simulink model "ATOM_simple_planning_2WS"  (R2026a)
settings: Solver=ode4  StopTime=15  FixedStep=0.01
model workspace (MAT data in the model file):
  vehicle.param.wheel_radius = 0.313
  vehicle.param.wheel_width = 0.235
  vehicle.param.wheel_base = 2
  vehicle.param.wheel_tread = 1.9
  vehicle.param.front_overhang = 0.46
  vehicle.param.rear_overhang = 0.46
  vehicle.param.left_overhang = 0.128
  vehicle.param.right_overhang = 0.128
  vehicle.param.vehicle_height = 1.8
  vehicle.param.max_steer_angle = 0.7
  vehicle.sim.vehicle_model_type = "DELAY_STEER_ACC_GEARED"
  vehicle.sim.initialize_source = "INITIAL_POSE_TOPIC"
  vehicle.sim.timer_sampling_time_ms = 25
  vehicle.sim.add_measurement_noise = 0
  vehicle.sim.vel_lim = 50
  vehicle.sim.vel_rate_lim = 7
  vehicle.sim.steer_lim = 1
  vehicle.sim.steer_rate_lim = 5
  vehicle.sim.acc_time_delay = 0.1
  vehicle.sim.acc_time_constant = 0.1
  vehicle.sim.steer_time_delay = 0.24
  vehicle.sim.steer_time_constant = 0.27
  vehicle.sim.x_stddev = 0.0001
  vehicle.sim.y_stddev = 0.0001
  vehicle.sim.steer_dead_band = 0
  vehicle.sim.steer_bias = 0
  vehicle.sim.debug_acc_scaling_factor = 1
  vehicle.sim.debug_steer_scaling_factor = 1
undefined symbols (not defined in the file or in its folder): planning_validator, stanley, velocity_smoother
(part 1 of 4)
settings Model: SimulationMode=accelerator  PacingRate=1000  Creator=andrea-ricetti  LastModifiedBy=andrea-ricetti

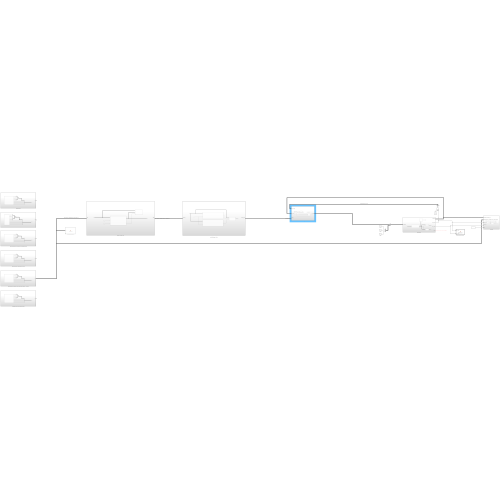
[thumbnail: Simulink's stored preview of the top-level diagram]
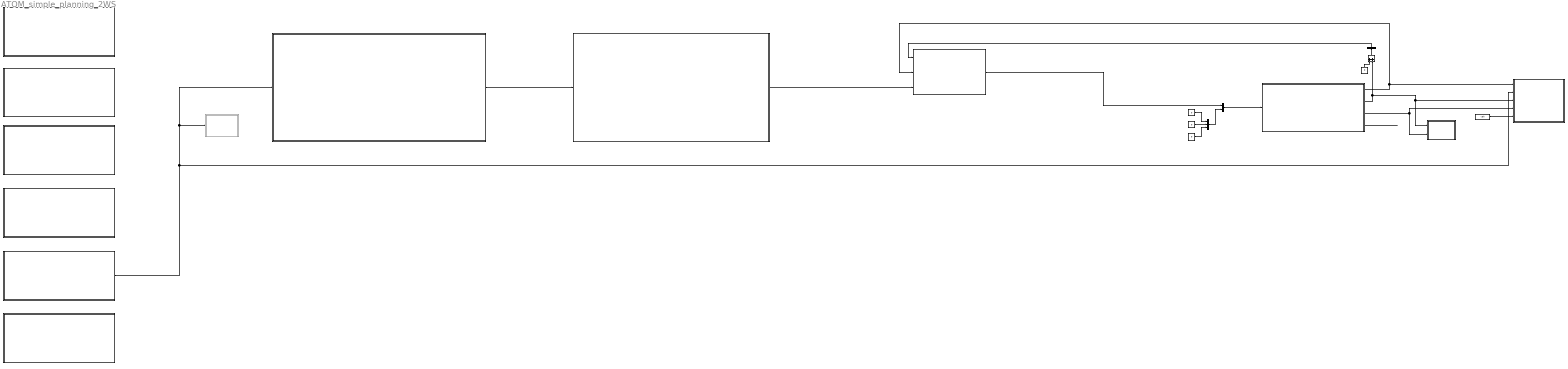
== system ATOM_simple_planning_2WS ==
  Add : Sum
  Bus Creator : BusCreator  Inputs=2  OutDataTypeStr=Bus: ControlCMDBus
      settings: InheritFromInputs=off
  Bus Creator2 : BusCreator  Inputs=3  OutDataTypeStr=Bus: LongitudinalBus
      settings: InheritFromInputs=off
  Bus Creator3 : BusCreator  Inputs=1  OutDataTypeStr=Bus: SteeringBus
      settings: InheritFromInputs=off
  Demanded trajectory generation: 90° left turn : Subsystem
  Demanded trajectory generation: 90° left turn critical for 2WS --> R = 2.5 m : Subsystem
  Demanded trajectory generation: Serpentine : Subsystem
  Demanded trajectory generation: Sinusoid 50m wavelength : Subsystem
  Demanded trajectory generation: smooth Parabola : Subsystem
  From Workspace1 : FromWorkspace  VariableName=veh
  Jerk : Constant  Value=0
  Lateral run() : Subsystem
  Plot demanded trajectory : MATLAB Function  Commented=on  TreatAsAtomicUnit=on
  Plot front/rear steer status : MATLAB Function  TreatAsAtomicUnit=on
  Plot vehicle : Subsystem
  Straight trajectory : Subsystem
  Vehicle Model : Subsystem
  acc : Constant  Value=0
  steer_bias : Constant  Value=0
  trajectory_checker plugin - planning_validator_node : Subsystem
  vel : Constant  Value=0
  velocity_smoother_node : Subsystem
  wires:
  Bus Creator2/1 -> Bus Creator/2
  vel/1 -> Bus Creator2/1
  acc/1 -> Bus Creator2/2
  Jerk/1 -> Bus Creator2/3
  Bus Creator/1 -> Vehicle Model/1(command)
  Vehicle Model/1(kinematic) -> Lateral run()/2(ego_pose), Plot vehicle/1(localization/kinematic_state)  "/localization/kinematic_state"
  Vehicle Model/3(steer_rear) -> Plot vehicle/4(steer_rear), Plot front/rear steer status/2(rear_steer)
  Demanded trajectory generation: 90° left turn critical for 2WS --> R = 2.5 m/1(traj) -> Plot vehicle/2(planning/scenario_planning/scenario_selector/trajectory), velocity_smoother_node/1(input), Plot demanded trajectory/1(traj)  "/planning/scenario_planning/scenario_selector/trajectory"
  Vehicle Model/4(accel) -> ?  "/localization/acceleration"
  velocity_smoother_node/1(output) -> trajectory_checker plugin - planning_validator_node/1(trajectory)  "/planning/scenario_planning/velocity_smoother/trajectory"
  trajectory_checker plugin - planning_validator_node/1(trajectory_out) -> Lateral run()/3(ref_traj)  "/planning/trajectory"
  Bus Creator3/1 -> Lateral run()/1(curr_steering)  "/vehicle/status/steering_status"
  Add/1 -> Bus Creator3/1
  steer_bias/1 -> Add/1
  Vehicle Model/2(steer_front) -> Add/2, Plot vehicle/3(steer_front), Plot front/rear steer status/1(front_steer)
  From Workspace1/1 -> Plot vehicle/5(veh)
  Lateral run()/1(ctrl_cmd) -> Bus Creator/1

== system ATOM_simple_planning_2WS/Demanded trajectory generation: 90° left turn ==
  Bus Creator3 : BusCreator  Inputs=3  OutDataTypeStr=Bus: PointBusN
  Bus Creator4 : BusCreator  Inputs=4  OutDataTypeStr=Bus: QuaternionBusN
  Bus Creator5 : BusCreator  Inputs=2  OutDataTypeStr=Bus: PoseBusN
      settings: InheritFromInputs=off
  Bus Creator6 : BusCreator  Inputs=7  OutDataTypeStr=Bus: TrajectoryDataBus
      settings: InheritFromInputs=off
  Trajectory Generator: 90° left turn : MATLAB Function  TreatAsAtomicUnit=on
  traj : Outport
  wires:
  Bus Creator6/1 -> traj/1
  Bus Creator3/1 -> Bus Creator5/1
  Trajectory Generator: 90° left turn/13(rear_wheel_angle_rad) -> Bus Creator6/7
  Bus Creator5/1 -> Bus Creator6/1
  Trajectory Generator: 90° left turn/8(longitudinal_velocity_mps) -> Bus Creator6/2
  Trajectory Generator: 90° left turn/3(z) -> Bus Creator3/3
  Trajectory Generator: 90° left turn/4(qx) -> Bus Creator4/1
  Trajectory Generator: 90° left turn/9(lateral_velocity_mps) -> Bus Creator6/3
  Trajectory Generator: 90° left turn/10(acceleration_mps2) -> Bus Creator6/4
  Trajectory Generator: 90° left turn/5(qy) -> Bus Creator4/2
  Trajectory Generator: 90° left turn/1(x) -> Bus Creator3/1
  Trajectory Generator: 90° left turn/2(y) -> Bus Creator3/2
  Trajectory Generator: 90° left turn/7(qw) -> Bus Creator4/4
  Trajectory Generator: 90° left turn/6(qz) -> Bus Creator4/3
  Trajectory Generator: 90° left turn/12(front_wheel_angle_rad) -> Bus Creator6/6
  Bus Creator4/1 -> Bus Creator5/2
  Trajectory Generator: 90° left turn/11(heading_rate_rps) -> Bus Creator6/5

== system ATOM_simple_planning_2WS/Demanded trajectory generation: 90° left turn critical for 2WS --> R = 2.5 m ==
  Bus Creator3 : BusCreator  Inputs=3  OutDataTypeStr=Bus: PointBusN
  Bus Creator4 : BusCreator  Inputs=4  OutDataTypeStr=Bus: QuaternionBusN
  Bus Creator5 : BusCreator  Inputs=2  OutDataTypeStr=Bus: PoseBusN
      settings: InheritFromInputs=off
  Bus Creator6 : BusCreator  Inputs=7  OutDataTypeStr=Bus: TrajectoryDataBus
      settings: InheritFromInputs=off
  Trajectory Generator: 90° left turn critical for 2WS : MATLAB Function  TreatAsAtomicUnit=on
  traj : Outport
  wires:
  Bus Creator6/1 -> traj/1
  Bus Creator3/1 -> Bus Creator5/1
  Trajectory Generator: 90° left turn critical for 2WS/13(rear_wheel_angle_rad) -> Bus Creator6/7
  Bus Creator5/1 -> Bus Creator6/1
  Trajectory Generator: 90° left turn critical for 2WS/8(longitudinal_velocity_mps) -> Bus Creator6/2
  Trajectory Generator: 90° left turn critical for 2WS/3(z) -> Bus Creator3/3
  Trajectory Generator: 90° left turn critical for 2WS/4(qx) -> Bus Creator4/1
  Trajectory Generator: 90° left turn critical for 2WS/9(lateral_velocity_mps) -> Bus Creator6/3
  Trajectory Generator: 90° left turn critical for 2WS/10(acceleration_mps2) -> Bus Creator6/4
  Trajectory Generator: 90° left turn critical for 2WS/5(qy) -> Bus Creator4/2
  Trajectory Generator: 90° left turn critical for 2WS/1(x) -> Bus Creator3/1
  Trajectory Generator: 90° left turn critical for 2WS/2(y) -> Bus Creator3/2
  Trajectory Generator: 90° left turn critical for 2WS/7(qw) -> Bus Creator4/4
  Trajectory Generator: 90° left turn critical for 2WS/6(qz) -> Bus Creator4/3
  Trajectory Generator: 90° left turn critical for 2WS/12(front_wheel_angle_rad) -> Bus Creator6/6
  Bus Creator4/1 -> Bus Creator5/2
  Trajectory Generator: 90° left turn critical for 2WS/11(heading_rate_rps) -> Bus Creator6/5

== system ATOM_simple_planning_2WS/Demanded trajectory generation: Serpentine ==
  Bus Creator3 : BusCreator  Inputs=3  OutDataTypeStr=Bus: PointBusN
  Bus Creator4 : BusCreator  Inputs=4  OutDataTypeStr=Bus: QuaternionBusN
  Bus Creator5 : BusCreator  Inputs=2  OutDataTypeStr=Bus: PoseBusN
      settings: InheritFromInputs=off
  Bus Creator6 : BusCreator  Inputs=7  OutDataTypeStr=Bus: TrajectoryDataBus
      settings: InheritFromInputs=off
  Trajectory Generator: 90° left turn critical for 2WS : MATLAB Function  TreatAsAtomicUnit=on
  traj : Outport
  wires:
  Bus Creator6/1 -> traj/1
  Bus Creator3/1 -> Bus Creator5/1
  Trajectory Generator: 90° left turn critical for 2WS/13(rear_wheel_angle_rad) -> Bus Creator6/7
  Bus Creator5/1 -> Bus Creator6/1
  Trajectory Generator: 90° left turn critical for 2WS/8(longitudinal_velocity_mps) -> Bus Creator6/2
  Trajectory Generator: 90° left turn critical for 2WS/3(z) -> Bus Creator3/3
  Trajectory Generator: 90° left turn critical for 2WS/4(qx) -> Bus Creator4/1
  Trajectory Generator: 90° left turn critical for 2WS/9(lateral_velocity_mps) -> Bus Creator6/3
  Trajectory Generator: 90° left turn critical for 2WS/10(acceleration_mps2) -> Bus Creator6/4
  Trajectory Generator: 90° left turn critical for 2WS/5(qy) -> Bus Creator4/2
  Trajectory Generator: 90° left turn critical for 2WS/1(x) -> Bus Creator3/1
  Trajectory Generator: 90° left turn critical for 2WS/2(y) -> Bus Creator3/2
  Trajectory Generator: 90° left turn critical for 2WS/7(qw) -> Bus Creator4/4
  Trajectory Generator: 90° left turn critical for 2WS/6(qz) -> Bus Creator4/3
  Trajectory Generator: 90° left turn critical for 2WS/12(front_wheel_angle_rad) -> Bus Creator6/6
  Bus Creator4/1 -> Bus Creator5/2
  Trajectory Generator: 90° left turn critical for 2WS/11(heading_rate_rps) -> Bus Creator6/5

== system ATOM_simple_planning_2WS/Demanded trajectory generation: Sinusoid 50m wavelength ==
  Bus Creator3 : BusCreator  Inputs=3  OutDataTypeStr=Bus: PointBusN
  Bus Creator4 : BusCreator  Inputs=4  OutDataTypeStr=Bus: QuaternionBusN
  Bus Creator5 : BusCreator  Inputs=2  OutDataTypeStr=Bus: PoseBusN
      settings: InheritFromInputs=off
  Bus Creator6 : BusCreator  Inputs=7  OutDataTypeStr=Bus: TrajectoryDataBus
      settings: InheritFromInputs=off
  Trajectory Generator: sinusoid : MATLAB Function  TreatAsAtomicUnit=on
  traj : Outport
  wires:
  Bus Creator6/1 -> traj/1
  Bus Creator3/1 -> Bus Creator5/1
  Trajectory Generator: sinusoid/13(rear_wheel_angle_rad) -> Bus Creator6/7
  Bus Creator5/1 -> Bus Creator6/1
  Trajectory Generator: sinusoid/8(longitudinal_velocity_mps) -> Bus Creator6/2
  Trajectory Generator: sinusoid/3(z) -> Bus Creator3/3
  Trajectory Generator: sinusoid/4(qx) -> Bus Creator4/1
  Trajectory Generator: sinusoid/9(lateral_velocity_mps) -> Bus Creator6/3
  Trajectory Generator: sinusoid/10(acceleration_mps2) -> Bus Creator6/4
  Trajectory Generator: sinusoid/5(qy) -> Bus Creator4/2
  Trajectory Generator: sinusoid/1(x) -> Bus Creator3/1
  Trajectory Generator: sinusoid/2(y) -> Bus Creator3/2
  Trajectory Generator: sinusoid/7(qw) -> Bus Creator4/4
  Trajectory Generator: sinusoid/6(qz) -> Bus Creator4/3
  Trajectory Generator: sinusoid/12(front_wheel_angle_rad) -> Bus Creator6/6
  Bus Creator4/1 -> Bus Creator5/2
  Trajectory Generator: sinusoid/11(heading_rate_rps) -> Bus Creator6/5

== system ATOM_simple_planning_2WS/Demanded trajectory generation: smooth Parabola ==
  Bus Creator3 : BusCreator  Inputs=3  OutDataTypeStr=Bus: PointBusN
  Bus Creator4 : BusCreator  Inputs=4  OutDataTypeStr=Bus: QuaternionBusN
  Bus Creator5 : BusCreator  Inputs=2  OutDataTypeStr=Bus: PoseBusN
      settings: InheritFromInputs=off
  Bus Creator6 : BusCreator  Inputs=7  OutDataTypeStr=Bus: TrajectoryDataBus
      settings: InheritFromInputs=off
  Smoothed Parabola trajectory : MATLAB Function  TreatAsAtomicUnit=on
  traj : Outport
  wires:
  Smoothed Parabola trajectory/5(qy) -> Bus Creator4/2
  Smoothed Parabola trajectory/6(qz) -> Bus Creator4/3
  Smoothed Parabola trajectory/11(heading_rate_rps) -> Bus Creator6/5
  Bus Creator5/1 -> Bus Creator6/1
  Bus Creator6/1 -> traj/1
  Smoothed Parabola trajectory/3(z) -> Bus Creator3/3
  Bus Creator4/1 -> Bus Creator5/2
  Smoothed Parabola trajectory/8(longitudinal_velocity_mps) -> Bus Creator6/2
  Smoothed Parabola trajectory/4(qx) -> Bus Creator4/1
  Smoothed Parabola trajectory/13(rear_wheel_angle_rad) -> Bus Creator6/7
  Smoothed Parabola trajectory/7(qw) -> Bus Creator4/4
  Smoothed Parabola trajectory/1(x) -> Bus Creator3/1
  Smoothed Parabola trajectory/2(y) -> Bus Creator3/2
  Bus Creator3/1 -> Bus Creator5/1
  Smoothed Parabola trajectory/12(front_wheel_angle_rad) -> Bus Creator6/6
  Smoothed Parabola trajectory/10(acceleration_mps2) -> Bus Creator6/4
  Smoothed Parabola trajectory/9(lateral_velocity_mps) -> Bus Creator6/3

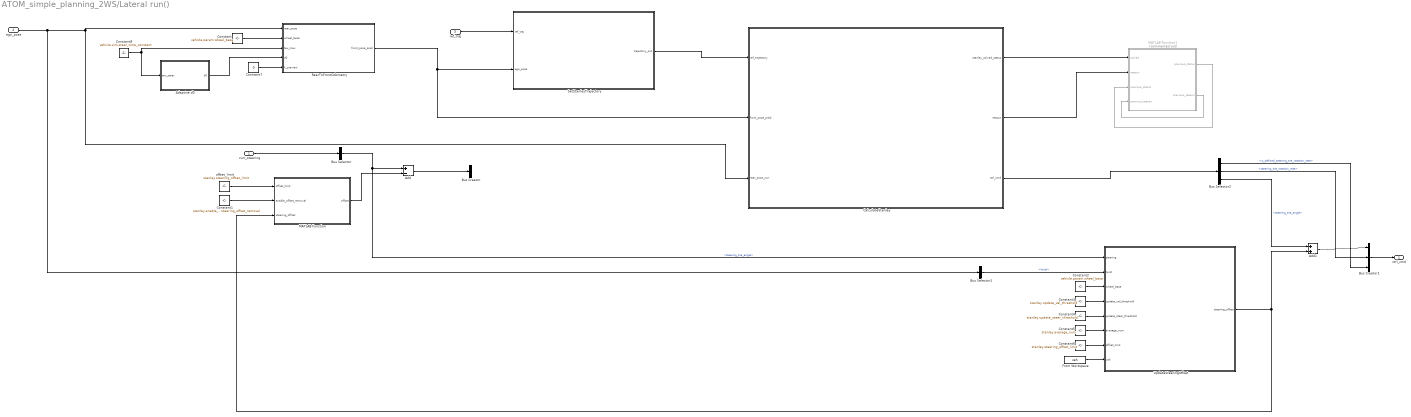
== system ATOM_simple_planning_2WS/Lateral run() ==
  curr_steering : Inport
  ego_pose : Inport  Port=2
  ref_traj : Inport  Port=3
  Adaptive d0 : MATLAB Function  TreatAsAtomicUnit=on
  Add : Sum  Inputs=+-
  Add1 : Sum
  Bus Creator : BusCreator  Inputs=1  OutDataTypeStr=Bus: SteeringBus
      settings: InheritFromInputs=off
  Bus Creator1 : BusCreator  Inputs=3  OutDataTypeStr=Bus: LateralBus
      settings: InheritFromInputs=off
  Bus Selector : BusSelector  OutputSignals=steering_tire_angle
  Bus Selector1 : BusSelector  OutputSignals=twist
  Bus Selector2 : BusSelector  OutputSignals=is_defined_steering_tire_rotation_rate,steering_tire_rotation_rate,steering_tire_angle
  CalculateStanley : Subsystem
  Constant : Constant  Value=vehicle.param.wheel_base
  Constant1 : Constant  Value=stanley.enable_auto_steering_offset_removal
  Constant2 : Constant  Value=vehicle.param.wheel_base
  Constant3 : Constant  Value=stanley.update_vel_threshold
  Constant4 : Constant  Value=stanley.update_steer_threshold
  Constant5 : Constant  Value=stanley.average_num
  Constant6 : Constant  Value=stanley.steering_offset_limit
  Constant7 : Constant  Value=0
  Constant8 : Constant  Value=vehicle.sim.steer_time_constant
  From Workspace : FromWorkspace  VariableName=veh
  MATLAB Function : MATLAB Function  TreatAsAtomicUnit=on
  MATLAB Function1 : MATLAB Function  Commented=on  TreatAsAtomicUnit=on
  RearToFrontOdometry : MATLAB Function  TreatAsAtomicUnit=on
  SetStanleyTrajectory : Subsystem
  UpdateSteeringOffset : MATLAB Function  TreatAsAtomicUnit=on
  offset_limit : Constant  Value=stanley.steering_offset_limit
  ctrl_cmd : Outport
  wires:
  ego_pose/1 -> Bus Selector1/1, CalculateStanley/3(rear_pose_curr), RearToFrontOdometry/1(rear_pose)
  Constant/1 -> RearToFrontOdometry/2(wheel_base)
  RearToFrontOdometry/1(front_pose_pred) -> CalculateStanley/2(front_pose_pred), SetStanleyTrajectory/2(ego_pose)
  curr_steering/1 -> Bus Selector/1
  offset_limit/1 -> MATLAB Function/1(offset_limit)
  Constant1/1 -> MATLAB Function/2(enable_offset_removal)
  Add/1 -> Bus Creator/1
  Bus Selector/1 -> UpdateSteeringOffset/1(steering), Add/1  "<steering_tire_angle>"
  ref_traj/1 -> SetStanleyTrajectory/1(ref_traj)
  SetStanleyTrajectory/1(trajectory_out) -> CalculateStanley/1(ref_trajectory)
  CalculateStanley/1(stanley_solved_status) -> MATLAB Function1/1(solved)
  CalculateStanley/2(reason) -> MATLAB Function1/2(reason)
  MATLAB Function1/2(previous_reason) -> MATLAB Function1/4("previous_reason ")
  MATLAB Function1/1(previous_status) -> MATLAB Function1/3("previous_status ")
  Bus Selector1/1 -> UpdateSteeringOffset/2(twist)  "<twist>"
  Constant2/1 -> UpdateSteeringOffset/3(wheel_base)
  Constant3/1 -> UpdateSteeringOffset/4(update_vel_threshold)
  Constant5/1 -> UpdateSteeringOffset/6(average_num)
  Constant4/1 -> UpdateSteeringOffset/5(update_steer_threshold)
  Constant6/1 -> UpdateSteeringOffset/7(offset_limit)
  From Workspace/1 -> UpdateSteeringOffset/8(veh)
  CalculateStanley/3(ctrl_cmd) -> Bus Selector2/1
  Bus Selector2/3 -> Add1/1  "<steering_tire_angle>"
  Add1/1 -> Bus Creator1/1
  Bus Selector2/1 -> Bus Creator1/3  "<is_defined_steering_tire_rotation_rate>"
  Bus Selector2/2 -> Bus Creator1/2  "<steering_tire_rotation_rate>"
  Bus Creator1/1 -> ctrl_cmd/1
  MATLAB Function/1(offset) -> Add/2
  UpdateSteeringOffset/1(steering_offset) -> MATLAB Function/3(steering_offset), Add1/2
  Constant8/1 -> Adaptive d0/1(tau_steer), RearToFrontOdometry/3(tau_max)
  Adaptive d0/1(d0) -> RearToFrontOdometry/4(d0)
  Constant7/1 -> RearToFrontOdometry/5(k_preview)

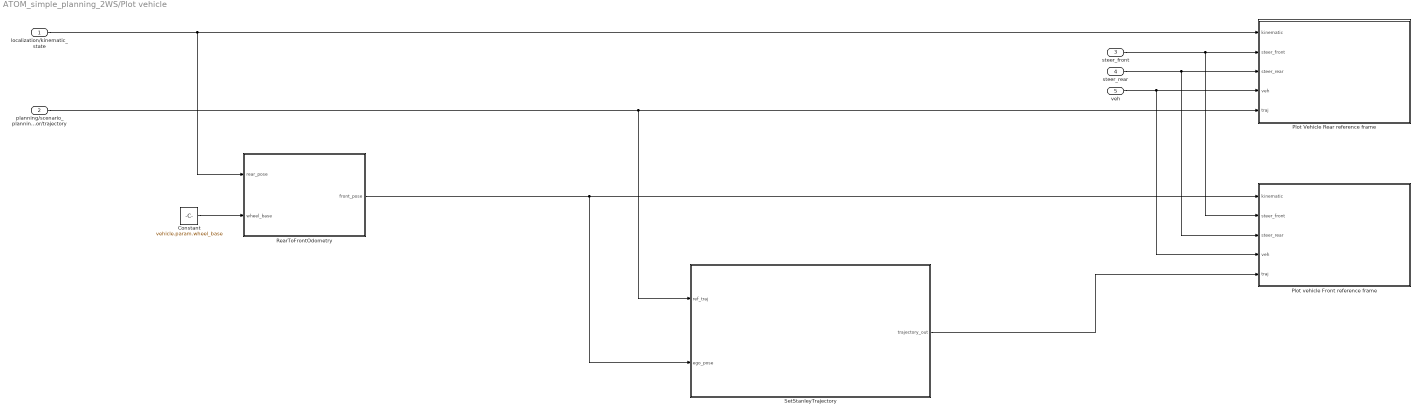
== system ATOM_simple_planning_2WS/Plot vehicle ==
  localization/kinematic_state : Inport
  planning/scenario_planning/scenario_selector/trajectory : Inport  Port=2
  steer_front : Inport  Port=3
  steer_rear : Inport  Port=4
  veh : Inport  Port=5
  Constant : Constant  Value=vehicle.param.wheel_base
  Plot Vehicle Rear reference frame : MATLAB Function  TreatAsAtomicUnit=on
  Plot vehicle Front reference frame : MATLAB Function  TreatAsAtomicUnit=on
  RearToFrontOdometry : MATLAB Function  TreatAsAtomicUnit=on
  SetStanleyTrajectory : Subsystem
  wires:
  steer_rear/1 -> Plot vehicle Front reference frame/3(steer_rear), Plot Vehicle Rear reference frame/3(steer_rear)
  veh/1 -> Plot vehicle Front reference frame/4(veh), Plot Vehicle Rear reference frame/4(veh)
  steer_front/1 -> Plot vehicle Front reference frame/2(steer_front), Plot Vehicle Rear reference frame/2(steer_front)
  Constant/1 -> RearToFrontOdometry/2(wheel_base)
  localization/kinematic_state/1 -> Plot Vehicle Rear reference frame/1(kinematic), RearToFrontOdometry/1(rear_pose)
  planning/scenario_planning/scenario_selector/trajectory/1 -> SetStanleyTrajectory/1(ref_traj), Plot Vehicle Rear reference frame/5(traj)
  RearToFrontOdometry/1(front_pose) -> SetStanleyTrajectory/2(ego_pose), Plot vehicle Front reference frame/1(kinematic)
  SetStanleyTrajectory/1(trajectory_out) -> Plot vehicle Front reference frame/5(traj)

== system ATOM_simple_planning_2WS/Straight trajectory ==
  Bus Creator3 : BusCreator  Inputs=3  OutDataTypeStr=Bus: PointBusN
  Bus Creator4 : BusCreator  Inputs=4  OutDataTypeStr=Bus: QuaternionBusN
  Bus Creator5 : BusCreator  Inputs=2  OutDataTypeStr=Bus: PoseBusN
      settings: InheritFromInputs=off
  Bus Creator6 : BusCreator  Inputs=7  OutDataTypeStr=Bus: TrajectoryDataBus
      settings: InheritFromInputs=off
  Trajectory Generator: straight : MATLAB Function  TreatAsAtomicUnit=on
  traj : Outport
  wires:
  Bus Creator6/1 -> traj/1
  Bus Creator3/1 -> Bus Creator5/1
  Trajectory Generator: straight/13(rear_wheel_angle_rad) -> Bus Creator6/7
  Bus Creator5/1 -> Bus Creator6/1
  Trajectory Generator: straight/8(longitudinal_velocity_mps) -> Bus Creator6/2
  Trajectory Generator: straight/3(z) -> Bus Creator3/3
  Trajectory Generator: straight/4(qx) -> Bus Creator4/1
  Trajectory Generator: straight/9(lateral_velocity_mps) -> Bus Creator6/3
  Trajectory Generator: straight/10(acceleration_mps2) -> Bus Creator6/4
  Trajectory Generator: straight/5(qy) -> Bus Creator4/2
  Trajectory Generator: straight/1(x) -> Bus Creator3/1
  Trajectory Generator: straight/2(y) -> Bus Creator3/2
  Trajectory Generator: straight/7(qw) -> Bus Creator4/4
  Trajectory Generator: straight/6(qz) -> Bus Creator4/3
  Trajectory Generator: straight/12(front_wheel_angle_rad) -> Bus Creator6/6
  Bus Creator4/1 -> Bus Creator5/2
  Trajectory Generator: straight/11(heading_rate_rps) -> Bus Creator6/5

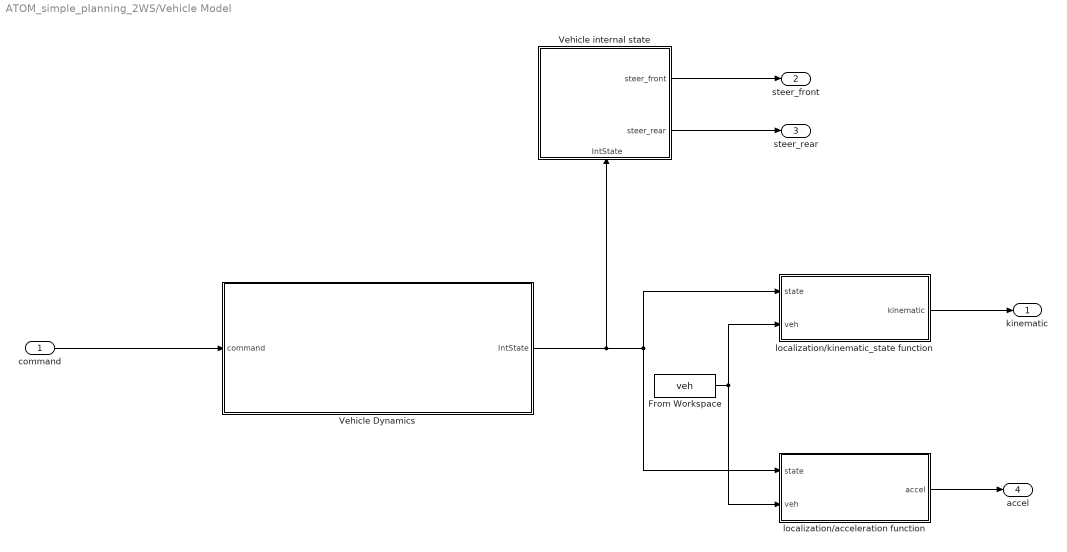
== system ATOM_simple_planning_2WS/Vehicle Model ==
  command : Inport
  From Workspace : FromWorkspace  VariableName=veh
  Vehicle Dynamics : Subsystem
  Vehicle internal state : Subsystem
      settings: PortSchema="{\"entries\":[{\"content\":{\"sides\":[{\"content\":{},\"type\":\"ConnectorPlacement.EquallySpacedRectSide\",\"uuid\":\"4a3566d2-c9ed-40f5-9383-803dea843249\"},{\"content\":{\"connectorIds\":[\"Out1\",\"Out2\"],\"side\":\"RIGHT\"},\"type\":\"ConnectorPlacement.EquallySpacedRectSide\",\"uuid\":\"38e6b545-4a7a-4953-bfc7-602e8f089057\"},{\"content\":{\"side\":\"TOP\"},\"type\":\"ConnectorPlacement.EquallySpacedRectSide\",\"uuid\":\"85394c7e-506c-43bc-a81e-512f61060685\"},{\"content\":{\"connectorIds\":[\"In1\"],\"side\":\"BOTTOM\"},\"type\":\"ConnectorPlacement.EquallySpacedRectSide\",\"uuid\":\"97da4b67-3c43-4e7d-b3d8-7f85e7f15c39\"}]},\"type\":\"ConnectorPlacement.EquallySpacedConnector\",\"uuid\":\"d0ddb274-13a9-46fc-8356-ac8c2bb4db82\"}],\"packageUris\":[\"http://schema.mathworks.com/mf0/Connector/R2020b\"],\"version\":\"1.0\"}"
  localization/acceleration function : MATLAB Function  TreatAsAtomicUnit=on
  localization/kinematic_state function : MATLAB Function  TreatAsAtomicUnit=on
  kinematic : Outport
  steer_front : Outport  Port=2
  steer_rear : Outport  Port=3
  accel : Outport  Port=4
  wires:
  From Workspace/1 -> localization/acceleration function/2(veh), localization/kinematic_state function/2(veh)
  Vehicle Dynamics/1(IntState) -> localization/kinematic_state function/1(state), localization/acceleration function/1(state), Vehicle internal state/1(IntState)
  Vehicle internal state/2(steer_rear) -> steer_rear/1
  command/1 -> Vehicle Dynamics/1(command)
  localization/kinematic_state function/1(kinematic) -> kinematic/1
  Vehicle internal state/1(steer_front) -> steer_front/1
  localization/acceleration function/1(accel) -> accel/1

== system ATOM_simple_planning_2WS/trajectory_checker plugin - planning_validator_node ==
  trajectory : Inport
  From Workspace2 : FromWorkspace  VariableName=veh
  HandleInvalidTrajectory - handling_type == default (case 0) : MATLAB Function  TreatAsAtomicUnit=on
  check_valid_steering : Subsystem
  check_valid_steering_rate : Subsystem
  trajectory_out : Outport
  wires:
  From Workspace2/1 -> check_valid_steering_rate/2(veh), check_valid_steering/2(veh)
  trajectory/1 -> check_valid_steering_rate/1(trajectory), HandleInvalidTrajectory - handling_type == default (case 0)/1(trajectory_in), check_valid_steering/1(trajectory)
  check_valid_steering/1(is_valid_steering) -> HandleInvalidTrajectory - handling_type == default (case 0)/2(is_valid_steering)
  check_valid_steering_rate/1(is_valid_steering_rate) -> HandleInvalidTrajectory - handling_type == default (case 0)/3(is_valid_steering_rate)
  HandleInvalidTrajectory - handling_type == default (case 0)/1(trajectory_out) -> trajectory_out/1

== system ATOM_simple_planning_2WS/velocity_smoother_node ==
  input : Inport
  ApplySteeringRateLimit - velocity_smoother_node : Subsystem
  MATLAB Function : MATLAB Function  Commented=on  TreatAsAtomicUnit=on
  input_points_interval [m] : Constant  OutDataTypeStr=double
  use_resampling == false : Constant  Value=0  OutDataTypeStr=boolean
  output : Outport
  wires:
  use_resampling == false/1 -> ApplySteeringRateLimit - velocity_smoother_node/2(use_resampling)
  ApplySteeringRateLimit - velocity_smoother_node/2(curvature) -> MATLAB Function/3(curvature)
  input/1 -> MATLAB Function/1(trajectory_input), ApplySteeringRateLimit - velocity_smoother_node/1(input From Trajecory topic --> TrajectoryPoints format)
  input_points_interval [m]/1 -> ApplySteeringRateLimit - velocity_smoother_node/3(input_points_interval)
  ApplySteeringRateLimit - velocity_smoother_node/1(output) -> output/1, MATLAB Function/2(trajectory_output)

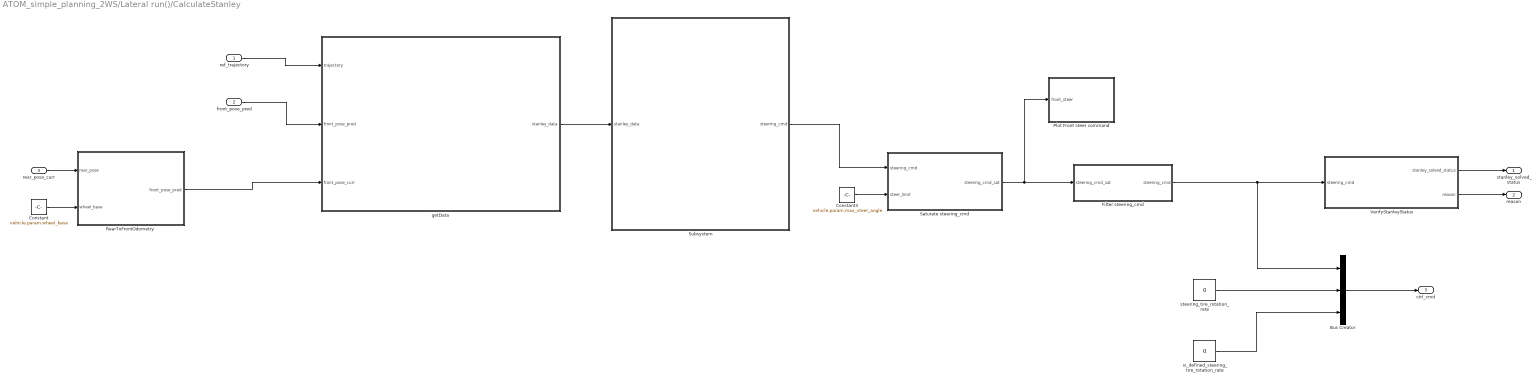
== system ATOM_simple_planning_2WS/Lateral run()/CalculateStanley ==
  ref_trajectory : Inport
  front_pose_pred : Inport  Port=2
  rear_pose_curr : Inport  Port=3
  Bus Creator : BusCreator  Inputs=3  OutDataTypeStr=Bus: LateralBus
      settings: InheritFromInputs=off
  Constant : Constant  Value=vehicle.param.wheel_base
  Constant3 : Constant  Value=vehicle.param.max_steer_angle
  Filter steering_cmd : MATLAB Function  TreatAsAtomicUnit=on
  Plot Front steer command : MATLAB Function  TreatAsAtomicUnit=on
  RearToFrontOdometry : MATLAB Function  TreatAsAtomicUnit=on
  Saturate steering_cmd : MATLAB Function  TreatAsAtomicUnit=on
  Subsystem : Subsystem
  VerifyStanleyStatus : MATLAB Function  TreatAsAtomicUnit=on
  getData : Subsystem
  is_defined_steering_tire_rotation_rate : Constant  Value=0  OutDataTypeStr=boolean
  steering_tire_rotation_rate : Constant  Value=0
  stanley_solved_status : Outport
  reason : Outport  Port=2
  ctrl_cmd : Outport  Port=3
  wires:
  ref_trajectory/1 -> getData/1(trajectory)
  front_pose_pred/1 -> getData/2(front_pose_pred)
  Constant3/1 -> Saturate steering_cmd/2(steer_limit)
  Saturate steering_cmd/1(steering_cmd_sat) -> Plot Front steer command/1(front_steer), Filter steering_cmd/1(steering_cmd_sat)
  Filter steering_cmd/1(steering_cmd) -> VerifyStanleyStatus/1(steering_cmd), Bus Creator/1
  steering_tire_rotation_rate/1 -> Bus Creator/2
  is_defined_steering_tire_rotation_rate/1 -> Bus Creator/3
  Bus Creator/1 -> ctrl_cmd/1
  VerifyStanleyStatus/1(stanley_solved_status) -> stanley_solved_status/1
  VerifyStanleyStatus/2(reason) -> reason/1
  getData/1(stanley_data) -> Subsystem/1(stanley_data)
  Subsystem/1(steering_cmd) -> Saturate steering_cmd/1(steering_cmd)
  Constant/1 -> RearToFrontOdometry/2(wheel_base)
  rear_pose_curr/1 -> RearToFrontOdometry/1(rear_pose)
  RearToFrontOdometry/1(front_pose_pred) -> getData/3(front_pose_curr)

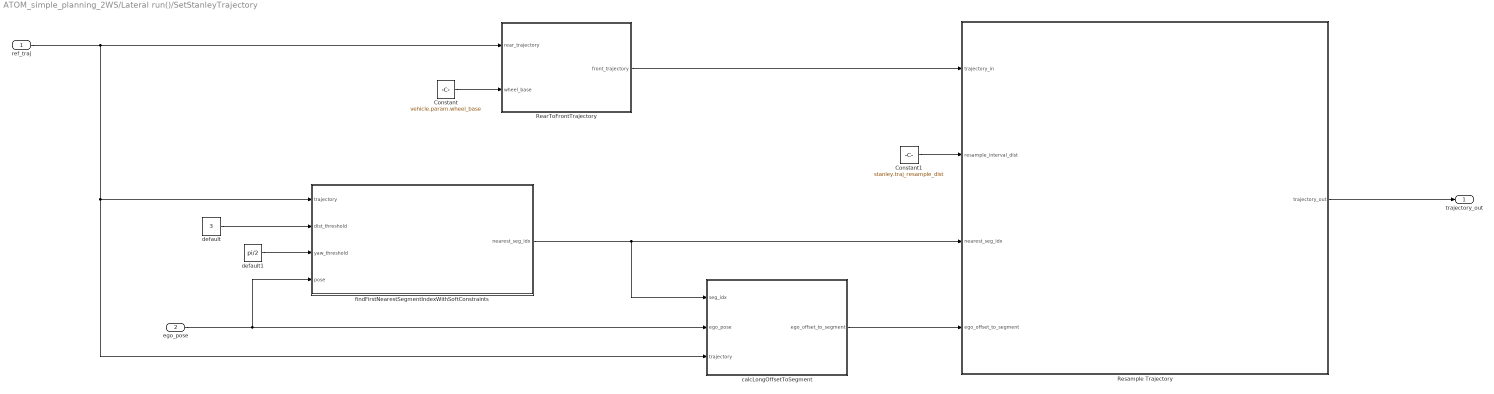
== system ATOM_simple_planning_2WS/Lateral run()/SetStanleyTrajectory ==
  ref_traj : Inport
  ego_pose : Inport  Port=2
  Constant : Constant  Value=vehicle.param.wheel_base
  Constant1 : Constant  Value=stanley.traj_resample_dist
  RearToFrontTrajectory : MATLAB Function  TreatAsAtomicUnit=on
  Resample Trajectory : MATLAB Function  TreatAsAtomicUnit=on
  calcLongOffsetToSegment : MATLAB Function  TreatAsAtomicUnit=on
  default : Constant  Value=3
  default1 : Constant  Value=pi/2
  findFirstNearestSegmentIndexWithSoftConstraints : MATLAB Function  TreatAsAtomicUnit=on
  trajectory_out : Outport
  wires:
  ref_traj/1 -> calcLongOffsetToSegment/3(trajectory), findFirstNearestSegmentIndexWithSoftConstraints/1(trajectory), RearToFrontTrajectory/1(rear_trajectory)
  Constant1/1 -> Resample Trajectory/2(resample_interval_dist)
  calcLongOffsetToSegment/1(ego_offset_to_segment) -> Resample Trajectory/4(ego_offset_to_segment)
  ego_pose/1 -> findFirstNearestSegmentIndexWithSoftConstraints/4(pose), calcLongOffsetToSegment/2(ego_pose)
  findFirstNearestSegmentIndexWithSoftConstraints/1(nearest_seg_idx) -> calcLongOffsetToSegment/1(seg_idx), Resample Trajectory/3(nearest_seg_idx)
  default/1 -> findFirstNearestSegmentIndexWithSoftConstraints/2(dist_threshold)
  default1/1 -> findFirstNearestSegmentIndexWithSoftConstraints/3(yaw_threshold)
  Resample Trajectory/1(trajectory_out) -> trajectory_out/1
  RearToFrontTrajectory/1(front_trajectory) -> Resample Trajectory/1(trajectory_in)
  Constant/1 -> RearToFrontTrajectory/2(wheel_base)

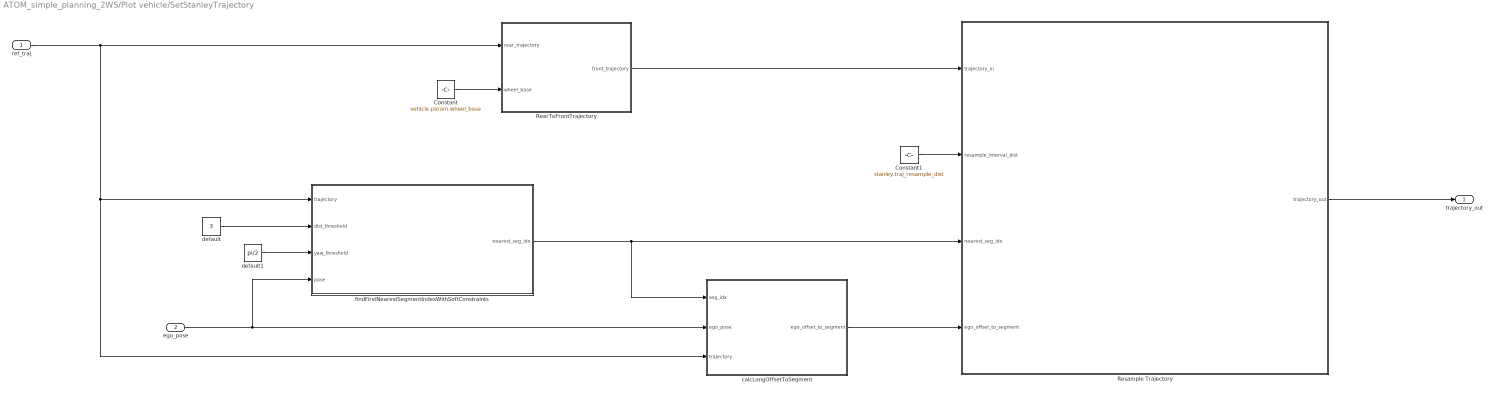
== system ATOM_simple_planning_2WS/Plot vehicle/SetStanleyTrajectory ==
  ref_traj : Inport
  ego_pose : Inport  Port=2
  Constant : Constant  Value=vehicle.param.wheel_base
  Constant1 : Constant  Value=stanley.traj_resample_dist
  RearToFrontTrajectory : MATLAB Function  TreatAsAtomicUnit=on
  Resample Trajectory : MATLAB Function  TreatAsAtomicUnit=on
  calcLongOffsetToSegment : MATLAB Function  TreatAsAtomicUnit=on
  default : Constant  Value=3
  default1 : Constant  Value=pi/2
  findFirstNearestSegmentIndexWithSoftConstraints : MATLAB Function  TreatAsAtomicUnit=on
  trajectory_out : Outport
  wires:
  ref_traj/1 -> calcLongOffsetToSegment/3(trajectory), findFirstNearestSegmentIndexWithSoftConstraints/1(trajectory), RearToFrontTrajectory/1(rear_trajectory)
  Constant1/1 -> Resample Trajectory/2(resample_interval_dist)
  calcLongOffsetToSegment/1(ego_offset_to_segment) -> Resample Trajectory/4(ego_offset_to_segment)
  ego_pose/1 -> findFirstNearestSegmentIndexWithSoftConstraints/4(pose), calcLongOffsetToSegment/2(ego_pose)
  findFirstNearestSegmentIndexWithSoftConstraints/1(nearest_seg_idx) -> calcLongOffsetToSegment/1(seg_idx), Resample Trajectory/3(nearest_seg_idx)
  default/1 -> findFirstNearestSegmentIndexWithSoftConstraints/2(dist_threshold)
  default1/1 -> findFirstNearestSegmentIndexWithSoftConstraints/3(yaw_threshold)
  Resample Trajectory/1(trajectory_out) -> trajectory_out/1
  RearToFrontTrajectory/1(front_trajectory) -> Resample Trajectory/1(trajectory_in)
  Constant/1 -> RearToFrontTrajectory/2(wheel_base)

== system ATOM_simple_planning_2WS/Vehicle Model/Vehicle Dynamics ==
  command : Inport
  From Workspace : FromWorkspace  VariableName=veh
  MATLAB Function : MATLAB Function  TreatAsAtomicUnit=on
  state integrator : Subsystem
  IntState : Outport
  wires:
  command/1 -> MATLAB Function/2(command)
  MATLAB Function/1(d_state) -> state integrator/1(d_state)  "d_state"
  state integrator/1(state) -> MATLAB Function/1(state), IntState/1
  From Workspace/1 -> MATLAB Function/3(veh)

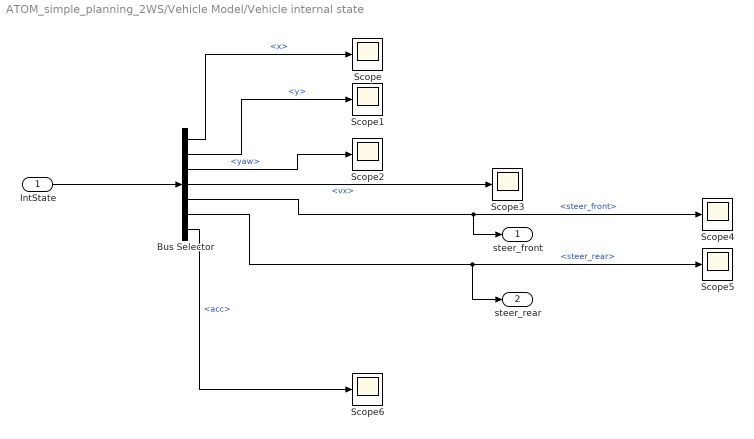
== system ATOM_simple_planning_2WS/Vehicle Model/Vehicle internal state ==
  IntState : Inport
  Bus Selector : BusSelector  OutputSignals=x,y,yaw,vx,steer_front,steer_rear,acc
  Scope{,1..6} (7 alike) : Scope
      Scope settings: ActiveDisplayYMinimum=-1  ActiveDisplayYMaximum=1
      Scope1 settings: ActiveDisplayYMinimum=-1  ActiveDisplayYMaximum=1
      Scope2 settings: ActiveDisplayYMinimum=-1  ActiveDisplayYMaximum=1  DataLoggingVariableName=ScopeData2
      Scope3 settings: ActiveDisplayYMinimum=-1  ActiveDisplayYMaximum=1  DataLoggingVariableName=ScopeData3
      Scope4 settings: ActiveDisplayYMinimum=-1  ActiveDisplayYMaximum=1  DataLoggingVariableName=ScopeData4
      Scope5 settings: ActiveDisplayYMinimum=-1  ActiveDisplayYMaximum=1  DataLoggingVariableName=ScopeData5
      Scope6 settings: ActiveDisplayYMinimum=-1  ActiveDisplayYMaximum=1  DataLoggingVariableName=ScopeData6
  steer_front : Outport
  steer_rear : Outport  Port=2
  wires:
  Bus Selector/2 -> Scope1/1  "<y>"
  Bus Selector/4 -> Scope3/1  "<vx>"
  Bus Selector/1 -> Scope/1  "<x>"
  Bus Selector/3 -> Scope2/1  "<yaw>"
  Bus Selector/7 -> Scope6/1  "<acc>"
  Bus Selector/5 -> steer_front/1, Scope4/1  "<steer_front>"
  Bus Selector/6 -> steer_rear/1, Scope5/1  "<steer_rear>"
  IntState/1 -> Bus Selector/1

== system ATOM_simple_planning_2WS/trajectory_checker plugin - planning_validator_node/check_valid_steering ==
  trajectory : Inport
  veh : Inport  Port=2
  CheckValidSteering : MATLAB Function  TreatAsAtomicUnit=on
  Constant : Constant  Value=planning_validator.steering.threshold
  calcMaxSteeringAngles : Subsystem
  is_valid_steering : Outport
  wires:
  calcMaxSteeringAngles/1(max_steering) -> CheckValidSteering/1(max_steering)
  calcMaxSteeringAngles/2(i) -> ?
  Constant/1 -> CheckValidSteering/2(steering_threshold)
  CheckValidSteering/1(is_valid_steering) -> is_valid_steering/1
  trajectory/1 -> calcMaxSteeringAngles/1(trajectory)
  veh/1 -> calcMaxSteeringAngles/2(veh)

== system ATOM_simple_planning_2WS/trajectory_checker plugin - planning_validator_node/check_valid_steering_rate ==
  trajectory : Inport
  veh : Inport  Port=2
  CheckValidSteeringRate : MATLAB Function  TreatAsAtomicUnit=on
  Constant : Constant  Value=planning_validator.steering_rate.threshold
  calcMaxSteeringRates : Subsystem
  is_valid_steering_rate : Outport
  wires:
  calcMaxSteeringRates/1(max_steering_rate) -> CheckValidSteeringRate/1(max_steering_rate)
  calcMaxSteeringRates/2(i) -> ?
  Constant/1 -> CheckValidSteeringRate/2(steering_rate_threshold)
  CheckValidSteeringRate/1(is_valid_steering_rate) -> is_valid_steering_rate/1
  trajectory/1 -> calcMaxSteeringRates/1(trajectory)
  veh/1 -> calcMaxSteeringRates/2(veh)

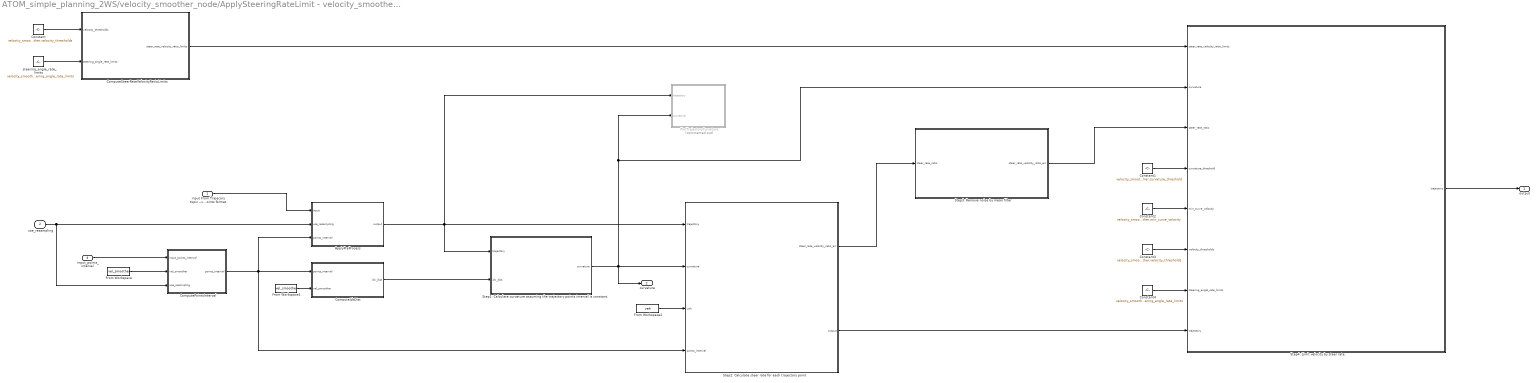
== system ATOM_simple_planning_2WS/velocity_smoother_node/ApplySteeringRateLimit - velocity_smoother_node ==
  input From Trajecory topic --> TrajectoryPoints format : Inport
  use_resampling : Inport  Port=2
  input_points_interval : Inport  Port=3
  ApplyPreProcess : MATLAB Function  TreatAsAtomicUnit=on
  ComputeIdxDist : MATLAB Function  TreatAsAtomicUnit=on
  ComputePointsInterval : MATLAB Function  TreatAsAtomicUnit=on
  ComputeSteerRateVelocityRatioLimits : MATLAB Function  TreatAsAtomicUnit=on
  Constant : Constant  Value=velocity_smoother.velocity_thresholds
  Constant1 : Constant  Value=velocity_smoother.curvature_threshold
  Constant2 : Constant  Value=velocity_smoother.min_curve_velocity
  Constant3 : Constant  Value=velocity_smoother.velocity_thresholds
  Constant4 : Constant  Value=velocity_smoother.steering_angle_rate_limits
  From Workspace : FromWorkspace  VariableName=vel_smoother
  From Workspace1 : FromWorkspace  VariableName=vel_smoother
  From Workspace2 : FromWorkspace  VariableName=veh
  PlotTrajectoryCurvature : MATLAB Function  Commented=on  TreatAsAtomicUnit=on
  Step1: Calculate curvature assuming the trajectory points interval is constant. : Subsystem
  Step2: Calculate steer rate for each trajectory point : Subsystem
  Step3: Remove noise by mean filter : Subsystem
  Step4: Limit velocity by steer rate. : Subsystem
  steering_angle_rate_limits : Constant  Value=velocity_smoother.steering_angle_rate_limits
  output : Outport
  curvature : Outport  Port=2
  wires:
  use_resampling/1 -> ApplyPreProcess/2(use_resempling), ComputePointsInterval/3(use_resampling)
  input From Trajecory topic --> TrajectoryPoints format/1 -> ApplyPreProcess/1(input)
  input_points_interval/1 -> ComputePointsInterval/1(input_points_interval)
  ComputePointsInterval/1(points_interval) -> Step2: Calculate steer rate for each trajectory point/4(points_interval), ComputeIdxDist/1(points_interval), ApplyPreProcess/3(points_interval)
  From Workspace/1 -> ComputePointsInterval/2(vel_smoother)
  From Workspace1/1 -> ComputeIdxDist/2(vel_smoother)
  ApplyPreProcess/1(output) -> PlotTrajectoryCurvature/1(trajectory), Step1: Calculate curvature assuming the trajectory points interval is constant./1(trajectory), Step2: Calculate steer rate for each trajectory point/1(trajectory)
  Step1: Calculate curvature assuming the trajectory points interval is constant./1(curvature) -> curvature/1, PlotTrajectoryCurvature/2(curvature), Step4: Limit velocity by steer rate./2(curvature), Step2: Calculate steer rate for each trajectory point/2(curvature)
  ComputeIdxDist/1(idx_dist) -> Step1: Calculate curvature assuming the trajectory points interval is constant./2(idx_dist)
  From Workspace2/1 -> Step2: Calculate steer rate for each trajectory point/3(veh)
  Step2: Calculate steer rate for each trajectory point/1(steer_rate_velocity_ratio_arr) -> Step3: Remove noise by mean filter/1(steer_rate_ratio)
  steering_angle_rate_limits/1 -> ComputeSteerRateVelocityRatioLimits/2(steering_angle_rate_limits)
  Constant/1 -> ComputeSteerRateVelocityRatioLimits/1(velocity_thresholds)
  ComputeSteerRateVelocityRatioLimits/1(steer_rate_velocity_ratio_limits) -> Step4: Limit velocity by steer rate./1(steer_rate_velocity_ratio_limits)
  Step3: Remove noise by mean filter/1(steer_rate_velocity_ratio_arr) -> Step4: Limit velocity by steer rate./3(steer_rate_ratio)
  Constant1/1 -> Step4: Limit velocity by steer rate./4(curvature_threshold)
  Constant2/1 -> Step4: Limit velocity by steer rate./5(min_curve_velocity)
  Constant3/1 -> Step4: Limit velocity by steer rate./6(velocity_thresholds)
  Constant4/1 -> Step4: Limit velocity by steer rate./7(steering_angle_rate_limits)
  Step2: Calculate steer rate for each trajectory point/2(output) -> Step4: Limit velocity by steer rate./8("trajectory ")
  Step4: Limit velocity by steer rate./1(trajectory) -> output/1

== system ATOM_simple_planning_2WS/Lateral run()/CalculateStanley/Subsystem ==
  stanley_data : Inport
  Constant : Constant  Value=0.8
  Constant1 : Constant  Value=stanley.k_soft
  Constant2 : Constant
  Constant4 : Constant  Value=vehicle.param.wheel_base
  calculateFrontSteer - Stanley : MATLAB Function  TreatAsAtomicUnit=on
  steering_cmd : Outport
  wires:
  Constant1/1 -> calculateFrontSteer - Stanley/3(k_soft)
  Constant/1 -> calculateFrontSteer - Stanley/2(k_gain)
  stanley_data/1 -> calculateFrontSteer - Stanley/1(stanley_data)
  calculateFrontSteer - Stanley/1(stanley_cmd) -> steering_cmd/1
  Constant4/1 -> calculateFrontSteer - Stanley/5(wheelbase)
  Constant2/1 -> calculateFrontSteer - Stanley/4(gain_4WS)

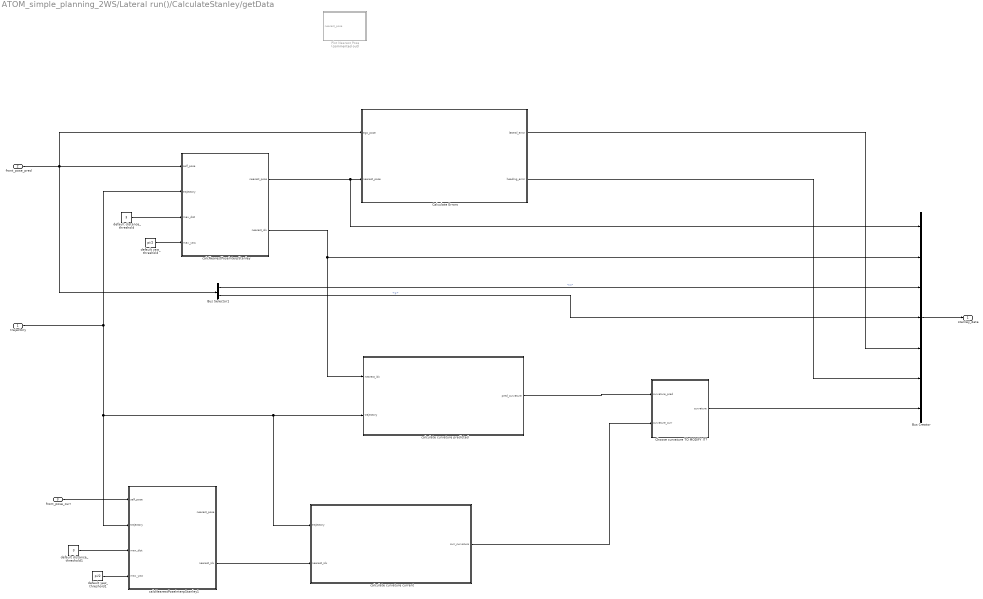
== system ATOM_simple_planning_2WS/Lateral run()/CalculateStanley/getData ==
  trajectory : Inport
  front_pose_pred : Inport  Port=2
  front_pose_curr : Inport  Port=3
  Bus Creator : BusCreator  Inputs=7  OutDataTypeStr=Bus: StanleyInputDataBus
      settings: InheritFromInputs=off
  Bus Selector1 : BusSelector  OutputSignals=twist.linear.x,twist.linear.y
  Calculate Errors : Subsystem
  Choose curvature TO MODIFY IT? : MATLAB Function  TreatAsAtomicUnit=on
  Plot Nearest Pose : MATLAB Function  Commented=on  TreatAsAtomicUnit=on
  calcNearestPoseInterpStanley : MATLAB Function  TreatAsAtomicUnit=on
  calcNearestPoseInterpStanley1 : MATLAB Function  TreatAsAtomicUnit=on
  calculate curvature current : Subsystem
  calculate curvature predicted : Subsystem
  default distance_threshold : Constant  Value=3
  default distance_threshold1 : Constant  Value=3
  default yaw_threshold : Constant  Value=pi/2
  default yaw_threshold1 : Constant  Value=pi/2
  stanley_data : Outport
  wires:
  default distance_threshold/1 -> calcNearestPoseInterpStanley/3(max_dist)
  default yaw_threshold/1 -> calcNearestPoseInterpStanley/4(max_yaw)
  front_pose_pred/1 -> Bus Selector1/1, Calculate Errors/1(ego_pose), calcNearestPoseInterpStanley/1(self_pose)
  calcNearestPoseInterpStanley/2(nearest_idx) -> calculate curvature predicted/1(nearest_idx), Bus Creator/2
  Bus Creator/1 -> stanley_data/1
  Bus Selector1/1 -> Bus Creator/3  "<x>"
  Calculate Errors/1(lateral_error) -> Bus Creator/5
  Calculate Errors/2(heading_error) -> Bus Creator/6
  calculate curvature predicted/1(pred_curvature) -> Choose curvature TO MODIFY IT?/1(curvature_pred)
  front_pose_curr/1 -> calcNearestPoseInterpStanley1/1(self_pose)
  default distance_threshold1/1 -> calcNearestPoseInterpStanley1/3(max_dist)
  default yaw_threshold1/1 -> calcNearestPoseInterpStanley1/4(max_yaw)
  calcNearestPoseInterpStanley1/2(nearest_idx) -> calculate curvature current/2(nearest_idx)
  trajectory/1 -> calcNearestPoseInterpStanley/2(trajectory), calcNearestPoseInterpStanley1/2(trajectory), calculate curvature current/1(trajectory), calculate curvature predicted/2(trajectory)
  calculate curvature current/1(curr_curvature) -> Choose curvature TO MODIFY IT?/2(curvature_curr)
  Choose curvature TO MODIFY IT?/1(curvature) -> Bus Creator/7
  calcNearestPoseInterpStanley/1(nearest_pose) -> Bus Creator/1, Calculate Errors/2(nearest_pose)
  Bus Selector1/2 -> Bus Creator/4  "<y>"

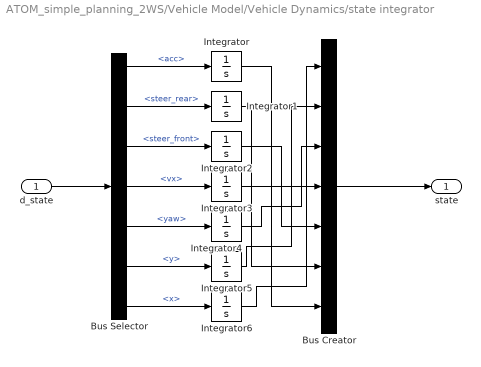
== system ATOM_simple_planning_2WS/Vehicle Model/Vehicle Dynamics/state integrator ==
  d_state : Inport
  Bus Creator : BusCreator  Inputs=7  OutDataTypeStr=Bus: VehicleInternalStateBus
      settings: InheritFromInputs=off
  Bus Selector : BusSelector  OutputSignals=acc,steer_rear,steer_front,vx,yaw,y,x
  Integrator{,1..2,4..6} (6 alike) : Integrator
  Integrator3 : Integrator  InitialCondition=4/3.6
  state : Outport
  wires:
  Integrator4/1 -> Bus Creator/3
  Integrator3/1 -> Bus Creator/4
  Integrator6/1 -> Bus Creator/1
  Bus Selector/4 -> Integrator3/1  "<vx>"
  Integrator1/1 -> Bus Creator/6
  Bus Creator/1 -> state/1
  Bus Selector/6 -> Integrator5/1  "<y>"
  Bus Selector/2 -> Integrator1/1  "<steer_rear>"
  Integrator5/1 -> Bus Creator/2
  Bus Selector/7 -> Integrator6/1  "<x>"
  Bus Selector/3 -> Integrator2/1  "<steer_front>"
  Bus Selector/1 -> Integrator/1  "<acc>"
  Integrator/1 -> Bus Creator/7
  Bus Selector/5 -> Integrator4/1  "<yaw>"
  d_state/1 -> Bus Selector/1
  Integrator2/1 -> Bus Creator/5

== system ATOM_simple_planning_2WS/trajectory_checker plugin - planning_validator_node/check_valid_steering/calcMaxSteeringAngles ==
  trajectory : Inport
  veh : Inport  Port=2
  DecideValIdx : MATLAB Function  TreatAsAtomicUnit=on
  GetAbsMaxValAndIdx front : MATLAB Function  TreatAsAtomicUnit=on
  GetAbsMaxValAndIdx rear : MATLAB Function  TreatAsAtomicUnit=on
  calcSteeringAngles : Subsystem
  max_steering : Outport
  i : Outport  Port=2
  wires:
  trajectory/1 -> calcSteeringAngles/1(trajectory)
  veh/1 -> calcSteeringAngles/2(veh)
  calcSteeringAngles/2(rear_steering_vector) -> GetAbsMaxValAndIdx rear/1(values)
  calcSteeringAngles/1(front_steering_vector) -> GetAbsMaxValAndIdx front/1(values)
  GetAbsMaxValAndIdx front/1(max_value) -> DecideValIdx/1(max_front)
  GetAbsMaxValAndIdx rear/2(max_index) -> DecideValIdx/4(idx_rear)
  GetAbsMaxValAndIdx rear/1(max_value) -> DecideValIdx/3(max_rear)
  GetAbsMaxValAndIdx front/2(max_index) -> DecideValIdx/2(idx_front)
  DecideValIdx/1(max_steering) -> max_steering/1
  DecideValIdx/2(max_index) -> i/1

== system ATOM_simple_planning_2WS/trajectory_checker plugin - planning_validator_node/check_valid_steering_rate/calcMaxSteeringRates ==
  trajectory : Inport
  veh : Inport  Port=2
  DecideValIdx : MATLAB Function  TreatAsAtomicUnit=on
  MATLAB Function : MATLAB Function  TreatAsAtomicUnit=on
  MATLAB Function1 : MATLAB Function  TreatAsAtomicUnit=on
  calcSteeringAngles : Subsystem
  max_steering_rate : Outport
  i : Outport  Port=2
  wires:
  trajectory/1 -> MATLAB Function1/1(trajectory), MATLAB Function/1(trajectory), calcSteeringAngles/1(trajectory)
  veh/1 -> calcSteeringAngles/2(veh)
  DecideValIdx/1(max_steering_rate) -> max_steering_rate/1
  DecideValIdx/2(max_index) -> i/1
  calcSteeringAngles/1(front_steering_vector) -> MATLAB Function/2(steering_vector)
  calcSteeringAngles/2(rear_steering_vector) -> MATLAB Function1/2(steering_vector)
  MATLAB Function/1(max_steering_rate) -> DecideValIdx/1(max_front)
  MATLAB Function/2(max_index) -> DecideValIdx/2(idx_front)
  MATLAB Function1/1(max_steering_rate) -> DecideValIdx/3(max_rear)
  MATLAB Function1/2(max_index) -> DecideValIdx/4(idx_rear)

== system ATOM_simple_planning_2WS/velocity_smoother_node/ApplySteeringRateLimit - velocity_smoother_node/Step1: Calculate curvature assuming the trajectory points interval is constant. ==
  trajectory : Inport
  idx_dist : Inport  Port=2
  CalcTrajectoryCurvature : MATLAB Function  TreatAsAtomicUnit=on
  curvature : Outport
  wires:
  idx_dist/1 -> CalcTrajectoryCurvature/2(idx_dist)
  CalcTrajectoryCurvature/1(curvature) -> curvature/1
  trajectory/1 -> CalcTrajectoryCurvature/1(trajectory)

== system ATOM_simple_planning_2WS/velocity_smoother_node/ApplySteeringRateLimit - velocity_smoother_node/Step2: Calculate steer rate for each trajectory point ==
  trajectory : Inport
  curvature : Inport  Port=2
  veh : Inport  Port=3
  points_interval : Inport  Port=4
  ComputeSteeringRate4WS : MATLAB Function  TreatAsAtomicUnit=on
  steer_rate_velocity_ratio_arr : Outport
  output : Outport  Port=2
  wires:
  curvature/1 -> ComputeSteeringRate4WS/2(curvature)
  trajectory/1 -> ComputeSteeringRate4WS/1(trajectory)
  points_interval/1 -> ComputeSteeringRate4WS/4(points_interval)
  veh/1 -> ComputeSteeringRate4WS/3(veh)
  ComputeSteeringRate4WS/1(steer_rate_velocity_ratio_arr) -> steer_rate_velocity_ratio_arr/1
  ComputeSteeringRate4WS/2(output) -> output/1

== system ATOM_simple_planning_2WS/velocity_smoother_node/ApplySteeringRateLimit - velocity_smoother_node/Step3: Remove noise by mean filter ==
  steer_rate_ratio : Inport
  MeanFilterSteeringRateRato : MATLAB Function  TreatAsAtomicUnit=on
  steer_rate_velocity_ratio_arr : Outport
  wires:
  steer_rate_ratio/1 -> MeanFilterSteeringRateRato/1(steer_rate_ratio)
  MeanFilterSteeringRateRato/1(steer_rate_velocity_ratio_arr) -> steer_rate_velocity_ratio_arr/1

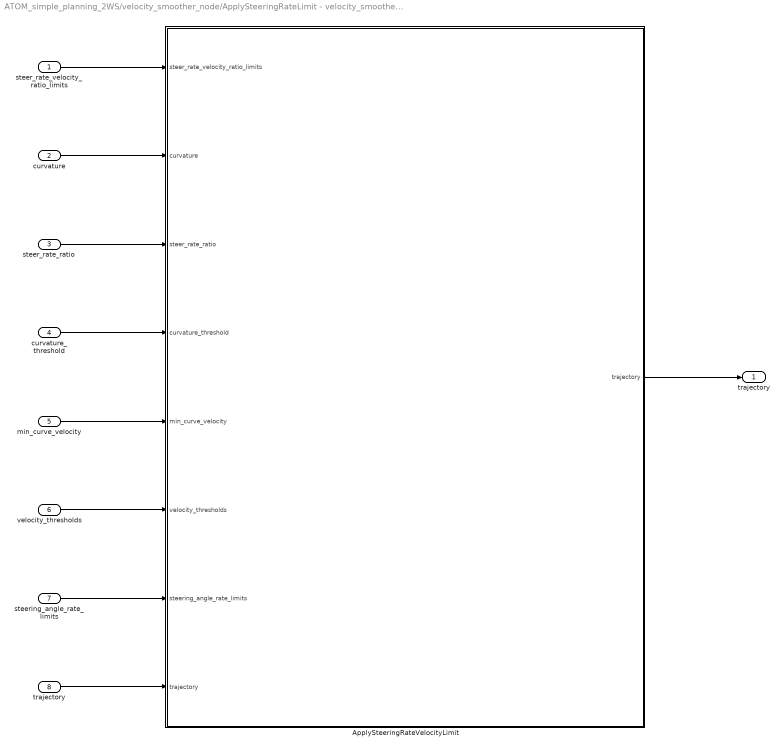
== system ATOM_simple_planning_2WS/velocity_smoother_node/ApplySteeringRateLimit - velocity_smoother_node/Step4: Limit velocity by steer rate. ==
  steer_rate_velocity_ratio_limits : Inport
  curvature : Inport  Port=2
  steer_rate_ratio : Inport  Port=3
  curvature_threshold : Inport  Port=4
  min_curve_velocity : Inport  Port=5
  velocity_thresholds : Inport  Port=6
  steering_angle_rate_limits : Inport  Port=7
  "trajectory " : Inport  Port=8
  ApplySteeringRateVelocityLimit : MATLAB Function  TreatAsAtomicUnit=on
  trajectory : Outport
  wires:
  velocity_thresholds/1 -> ApplySteeringRateVelocityLimit/6(velocity_thresholds)
  ApplySteeringRateVelocityLimit/1(trajectory) -> trajectory/1
  "trajectory "/1 -> ApplySteeringRateVelocityLimit/8("trajectory ")
  steer_rate_velocity_ratio_limits/1 -> ApplySteeringRateVelocityLimit/1(steer_rate_velocity_ratio_limits)
  curvature/1 -> ApplySteeringRateVelocityLimit/2(curvature)
  steer_rate_ratio/1 -> ApplySteeringRateVelocityLimit/3(steer_rate_ratio)
  steering_angle_rate_limits/1 -> ApplySteeringRateVelocityLimit/7(steering_angle_rate_limits)
  curvature_threshold/1 -> ApplySteeringRateVelocityLimit/4(curvature_threshold)
  min_curve_velocity/1 -> ApplySteeringRateVelocityLimit/5(min_curve_velocity)

== system ATOM_simple_planning_2WS/Lateral run()/CalculateStanley/getData/Calculate Errors ==
  ego_pose : Inport
  nearest_pose : Inport  Port=2
  Plot Stanley Errors : MATLAB Function  TreatAsAtomicUnit=on
  calcLateralErrorStanley : MATLAB Function  TreatAsAtomicUnit=on
  calcYawErrorStanley : MATLAB Function  TreatAsAtomicUnit=on
  lateral_error : Outport
  heading_error : Outport  Port=2
  wires:
  nearest_pose/1 -> calcYawErrorStanley/2(nearest_pose), calcLateralErrorStanley/2(nearest_pose)
  ego_pose/1 -> calcLateralErrorStanley/1(ego_pose), calcYawErrorStanley/1(ego_pose)
  calcYawErrorStanley/1(yaw_err) -> heading_error/1, Plot Stanley Errors/2(heading_error)
  calcLateralErrorStanley/1(lateral_error) -> lateral_error/1, Plot Stanley Errors/1(lateral_error)

== system ATOM_simple_planning_2WS/Lateral run()/CalculateStanley/getData/calculate curvature current ==
  trajectory : Inport
  nearest_idx : Inport  Port=2
  CalcTrajectoryCurvature : MATLAB Function  TreatAsAtomicUnit=on
  ComputeIdxDist : MATLAB Function  TreatAsAtomicUnit=on
  ComputePointsInterval : MATLAB Function  TreatAsAtomicUnit=on
  From Workspace : FromWorkspace  VariableName=vel_smoother
  From Workspace1 : FromWorkspace  VariableName=vel_smoother
  input_points_interval [m] : Constant  OutDataTypeStr=double
  use_resampling == false : Constant  Value=0  OutDataTypeStr=boolean
  curr_curvature : Outport
  wires:
  From Workspace1/1 -> ComputeIdxDist/2(vel_smoother)
  CalcTrajectoryCurvature/1(curvature) -> curr_curvature/1
  use_resampling == false/1 -> ComputePointsInterval/3(use_resampling)
  ComputePointsInterval/1(points_interval) -> ComputeIdxDist/1(points_interval)
  From Workspace/1 -> ComputePointsInterval/2(vel_smoother)
  input_points_interval [m]/1 -> ComputePointsInterval/1(input_points_interval)
  trajectory/1 -> CalcTrajectoryCurvature/1(trajectory)
  ComputeIdxDist/1(idx_dist) -> CalcTrajectoryCurvature/3(idx_dist)
  nearest_idx/1 -> CalcTrajectoryCurvature/2(nearest_idx)

== system ATOM_simple_planning_2WS/Lateral run()/CalculateStanley/getData/calculate curvature predicted ==
  nearest_idx : Inport
  trajectory : Inport  Port=2
  CalcTrajectoryCurvature : MATLAB Function  TreatAsAtomicUnit=on
  ComputeIdxDist : MATLAB Function  TreatAsAtomicUnit=on
  ComputePointsInterval : MATLAB Function  TreatAsAtomicUnit=on
  From Workspace : FromWorkspace  VariableName=vel_smoother
  From Workspace1 : FromWorkspace  VariableName=vel_smoother
  input_points_interval [m] : Constant  OutDataTypeStr=double
  use_resampling == false : Constant  Value=0  OutDataTypeStr=boolean
  pred_curvature : Outport
  wires:
  From Workspace1/1 -> ComputeIdxDist/2(vel_smoother)
  CalcTrajectoryCurvature/1(curvature) -> pred_curvature/1
  use_resampling == false/1 -> ComputePointsInterval/3(use_resampling)
  ComputePointsInterval/1(points_interval) -> ComputeIdxDist/1(points_interval)
  From Workspace/1 -> ComputePointsInterval/2(vel_smoother)
  input_points_interval [m]/1 -> ComputePointsInterval/1(input_points_interval)
  trajectory/1 -> CalcTrajectoryCurvature/1(trajectory)
  ComputeIdxDist/1(idx_dist) -> CalcTrajectoryCurvature/3(idx_dist)
  nearest_idx/1 -> CalcTrajectoryCurvature/2(nearest_idx)

== system ATOM_simple_planning_2WS/trajectory_checker plugin - planning_validator_node/check_valid_steering/calcMaxSteeringAngles/calcSteeringAngles ==
  trajectory : Inport
  veh : Inport  Port=2
  calcCurvature : MATLAB Function  TreatAsAtomicUnit=on
  steering_vector calculation : MATLAB Function  TreatAsAtomicUnit=on
  front_steering_vector : Outport
  rear_steering_vector : Outport  Port=2
  wires:
  steering_vector calculation/2(rear_steering_vector) -> rear_steering_vector/1
  veh/1 -> steering_vector calculation/2(veh)
  trajectory/1 -> calcCurvature/1(trajectory)
  calcCurvature/1(curvature_vector) -> steering_vector calculation/1(curvature)
  steering_vector calculation/1(front_steering_vector) -> front_steering_vector/1

== system ATOM_simple_planning_2WS/trajectory_checker plugin - planning_validator_node/check_valid_steering_rate/calcMaxSteeringRates/calcSteeringAngles ==
  trajectory : Inport
  veh : Inport  Port=2
  calcCurvature : MATLAB Function  TreatAsAtomicUnit=on
  steering_vector calculation : MATLAB Function  TreatAsAtomicUnit=on
  front_steering_vector : Outport
  rear_steering_vector : Outport  Port=2
  wires:
  steering_vector calculation/2(rear_steering_vector) -> rear_steering_vector/1
  veh/1 -> steering_vector calculation/2(veh)
  trajectory/1 -> calcCurvature/1(trajectory)
  calcCurvature/1(curvature_vector) -> steering_vector calculation/1(curvature)
  steering_vector calculation/1(front_steering_vector) -> front_steering_vector/1
